simulink model "hw2_q4"  (R2018b)
settings: Solver=VariableStepAuto  StartTime=0.0  StopTime=20  RelTol=1e-3
settings Model: Creator=Sazgar Shargh  LastModifiedBy=Sazgar Shargh

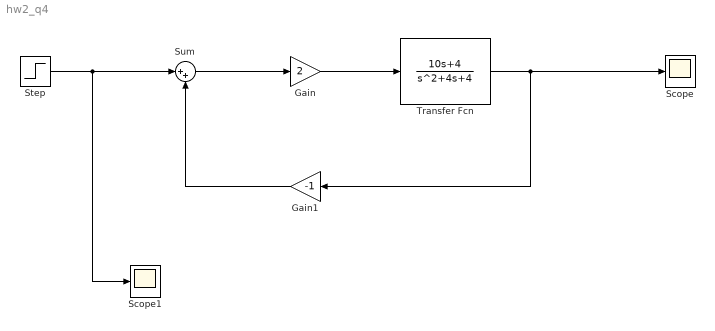
== system hw2_q4 ==
  Gain : Gain  Gain=2
  Gain1 : Gain  Gain=-1
  Scope : Scope
  Scope1 : Scope
  Step : Step  Time=0.0001  SampleTime=5
  Sum : Sum  Inputs=|++
  Transfer Fcn : TransferFcn  Numerator=[10 4]  Denominator=[1 4 4]
  wires:
  Transfer Fcn/1 -> Gain1/1, Scope/1
  Gain/1 -> Transfer Fcn/1
  Sum/1 -> Gain/1
  Step/1 -> Scope1/1, Sum/1
  Gain1/1 -> Sum/2
